simulink model "pid_vs_fuzzy_controllers_cesar"  (R2022b)
settings: Solver=VariableStepAuto  StartTime=0.0  StopTime=61  RelTol=1e-3
libraries: fuzblock x1, slpidlib x1
settings Model: Creator=cesarasa  LastModifiedBy=cesarasa

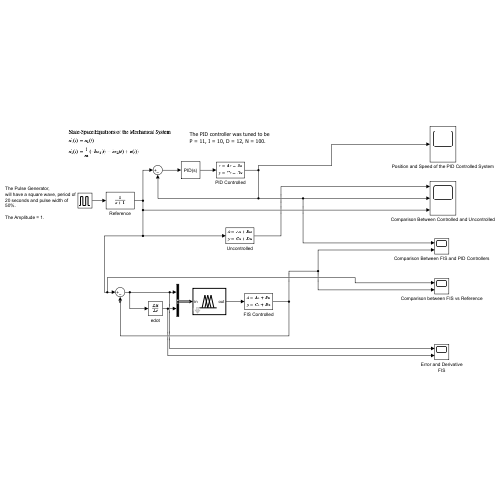
[thumbnail: Simulink's stored preview of the top-level diagram]
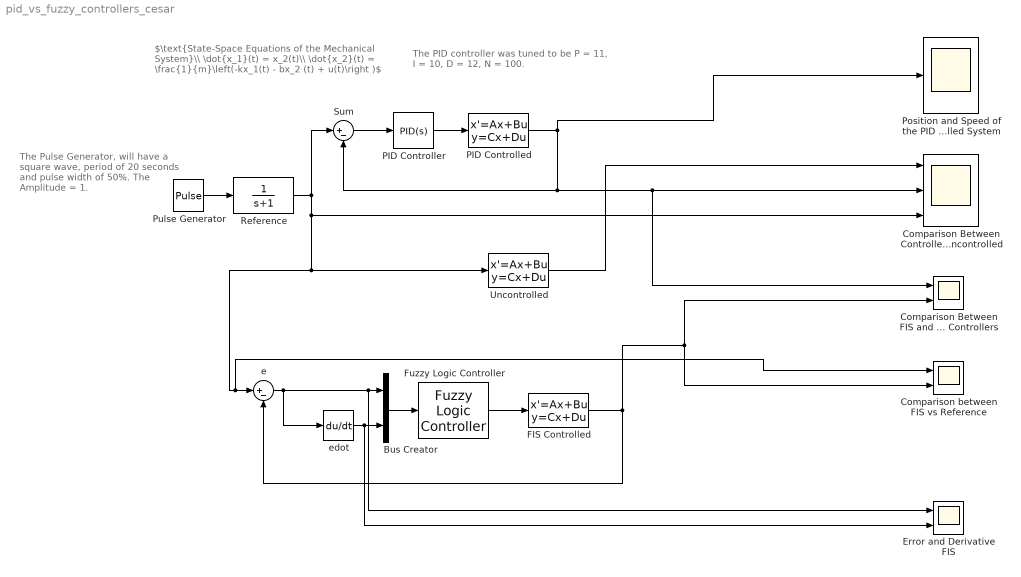
== system pid_vs_fuzzy_controllers_cesar ==
  note: The PID controller was tuned to be
      | P = 11, I = 10, D = 12, N = 100.
  note: The Pulse Generator,
      | will have a square wave, period of 20 seconds and pulse width of 50%.
      |
      | The Amplitude = 1.
  note: $\text{State-Space Equations of the Mechanical System}\\ \dot{x_1}(t) = x_2(t)\\ \dot{x_2}(t) = \frac{1}{m}\left(-kx_1(t) - bx_2 (t) + u(t)\right )$
  Bus Creator : BusCreator  Inputs=2
  Comparison Between Controlled and Uncontrolled : Scope  NumInputPorts=3
  Comparison Between FIS and PID Controllers : Scope  NumInputPorts=2
  Comparison between FIS vs Reference : Scope  NumInputPorts=2
  Error and Derivative FIS : Scope  NumInputPorts=2
  FIS Controlled : StateSpace  A=[0 1; -1 -1]  B=[0 1]'  C=[1 0]  D=0  InitialCondition=0  ParameterTunability=Unconstrained
  Fuzzy Logic Controller : fuzblock/Fuzzy Logic  Controller  FIS='controller_fuzzy.fis'  OutputSampleNumber=101  DataType=double  FuzzifiedInputs=off  RuleFiringStrengths=off  RuleOutputs=off  AggregatedOutputs=off  SimulateUsing=Code generation  OutOfRangeInputValueMessage=warning  NoRuleFiredMessage=warning  EmptyOutputFuzzySetMessage=warning
  PID Controlled : StateSpace  A=[0 1; -1 -1]  B=[0 1; 0 0]'  C=[1 0; 0 1 ]  D=[0 0;0 0]  InitialCondition=0  ParameterTunability=Unconstrained
  PID Controller : slpidlib/PID Controller  Controller=PID  Form=Parallel  TimeDomain=Continuous-time  UseExternalTs=off  SampleTime=-1  IntegratorMethod=Forward Euler  FilterMethod=Forward Euler  ControllerParametersSource=internal  P=11  I=10  UseKiTs=off  D=12  N=100  UseFilter=on  TunerSelectOption=Transfer Function Based (PID Tuner App)  ZeroCross=off  InitialConditionSource=internal  InitialConditionForIntegrator=0  InitialConditionForFilter=0  DifferentiatorICPrevScaledInput=0  ExternalReset=none  TrackingMode=off  Kt=1  LimitOutput=off  SatLimitsSource=internal  UpperSaturationLimit=inf  LowerSaturationLimit=-inf  LinearizeAsGain=on  AntiWindupMode=none  Kb=1  LimitIntegrator=off  UpperIntegratorSaturationLimit=inf  LowerIntegratorSaturationLimit=-inf  POutMin=[]  POutMax=[]  IOutMin=[]  IOutMax=[]  DOutMin=[]  DOutMax=[]  NOutMin=[]  NOutMax=[]  SumOutMin=[]  SumOutMax=[]  SaturationOutMin=[]  SaturationOutMax=[]  PParamMin=[]  PParamMax=[]  IParamMin=[]  IParamMax=[]  DParamMin=[]  DParamMax=[]  NParamMin=[]  NParamMax=[]  KbParamMin=[]  KbParamMax=[]  KtParamMin=[]  KtParamMax=[]  KbOutMin=[]  KbOutMax=[]  KtOutMin=[]  KtOutMax=[]  IntegratorOutMin=[]  IntegratorOutMax=[]  FilterOutMin=[]  FilterOutMax=[]  SumI1OutMin=[]  SumI1OutMax=[]  SumI2OutMin=[]  SumI2OutMax=[]  SumI3OutMin=[]  SumI3OutMax=[]  SumI4OutMin=[]  SumI4OutMax=[]  SumDOutMin=[]  SumDOutMax=[]  DifferentiatorOutMin=[]  DifferentiatorOutMax=[]  FilterDiffOutCoefMin=[]  FilterDiffOutCoefMax=[]  ReciprocalOutMin=[]  ReciprocalOutMax=[]  SumDenOutMin=[]  SumDenOutMax=[]  SumNumOutMin=[]  SumNumOutMax=[]  DivideOutMin=[]  DivideOutMax=[]  UdiffTsProdOutMin=[]  UdiffTsProdOutMax=[]  NTsProdOutMin=[]  NTsProdOutMax=[]  UintegralTsProdOutMin=[]  UintegralTsProdOutMax=[]  UngainTsProdOutMin=[]  UngainTsProdOutMax=[]  ClampingZeroOutDataTypeStr=Inherit: Inherit via back propagation  ClampingZeroOutMin=[]  ClampingZeroOutMax=[]  FilterDenConstantOutDataTypeStr=Inherit: Inherit via back propagation  FilterDenConstantOutMin=[]  FilterDenConstantOutMax=[]  PCopyOutDataTypeStr=Inherit: Inherit via back propagation  PCopyOutMin=[]  PCopyOutMax=[]  NCopyOutDataTypeStr=Inherit: Inherit via back propagation  NCopyOutMin=[]  NCopyOutMax=[]  IntegratorContinuousStateAttributes=''  IntegratorStateMustResolveToSignalObject=off  IntegratorRTWStateStorageClass=Auto  FilterContinuousStateAttributes=''  FilterStateMustResolveToSignalObject=off  FilterRTWStateStorageClass=Auto  ParallelPVariant=InternalParameters  IdealPVariant=Disabled  IVariant=InternalParameters  DVariant=InternalParameters  IntegratorVariant=Continuous  SatVariant=Disabled  AWVariant=Passthrough  PCopyVariant=Disabled  TRVariant=Disabled  FdbkBlocksVariant=Forward  IdealPFdbkVariant=Disabled  SatFdbkVariant=Disabled  DerivativeFilterVariant=ContFilter  NVariant=InternalParameters  NCopyVariant=Disabled  FilterICVariant=InternalICsFilter  IntegratorICVariant=InternalICs  ExternalResetVariant=Disabled  TRSumVariant=Passthrough  SumFdbkVariant=Disabled  SumVariant=Sum_PID  TsampFilterVariant=InternalTs  TsampNgainVariant=Passthrough  TsampIntegralVariant=Passthrough  ExternalSaturationOutDataTypeStr=Inherit: Same as second input
  Position and Speed of the PID Controlled System : Scope
  Pulse Generator : DiscretePulseGenerator  PulseType=Time based  Period=30  PulseWidth=50  PhaseDelay=1
  Reference : TransferFcn  Denominator=[1 1]
  Sum : Sum  Inputs=|+-
  Uncontrolled : StateSpace  A=[0 1; -1 -1]  B=[0 1]'  C=[1 0]  D=0  InitialCondition=0  ParameterTunability=Unconstrained
  e : Sum  Inputs=|+-
  edot : Derivative
  wires:
  Uncontrolled/1 -> Comparison Between Controlled and Uncontrolled/1
  PID Controlled/1 -> Comparison Between FIS and PID Controllers/1, Comparison Between Controlled and Uncontrolled/2, Sum/2, Position and Speed of the PID Controlled System/1
  PID Controller/1 -> PID Controlled/1
  Pulse Generator/1 -> Reference/1
  Sum/1 -> PID Controller/1
  Reference/1 -> Uncontrolled/1, Comparison between FIS vs Reference/1, e/1, Comparison Between Controlled and Uncontrolled/3, Sum/1
  Fuzzy Logic Controller/1 -> FIS Controlled/1
  FIS Controlled/1 -> Comparison Between FIS and PID Controllers/2, Comparison between FIS vs Reference/2, e/2
  e/1 -> edot/1, Error and Derivative FIS/1, Bus Creator/1
  Bus Creator/1 -> Fuzzy Logic Controller/1
  edot/1 -> Error and Derivative FIS/2, Bus Creator/2
